simulink model "Full_Model_R1"  (R2013a)
settings: Solver=ode45  StartTime=0.0  StopTime=sim_length  MaxStep=1e-4  RelTol=1e-3
values from neighbouring files (symbols this model uses):
  K = [1 1.29039130411 0.306791381023]    [Yaw_Controller_SS_Data.mat]
  Kp_Height = 3.52780854887    [Height_Controller.mat]
undefined symbols (not defined in the file or in its folder): B, D, F_yIntercept, g, I_Phi, I_Psi, I_Theta, J, Kf, Kw, L, Mass, Motor_TimeConstant, Nbar1, Phi_IC, Pitch_Setpoint, Psi_IC, PWM_LimHigher, PWM_LimLower, Roll_Setpoint, Speed_yIntercept, T_I_Height, Theta_IC, Yaw_Setpoint
libraries: simulink x4
settings Model: Creator=Ross  LastModifiedBy=Ross

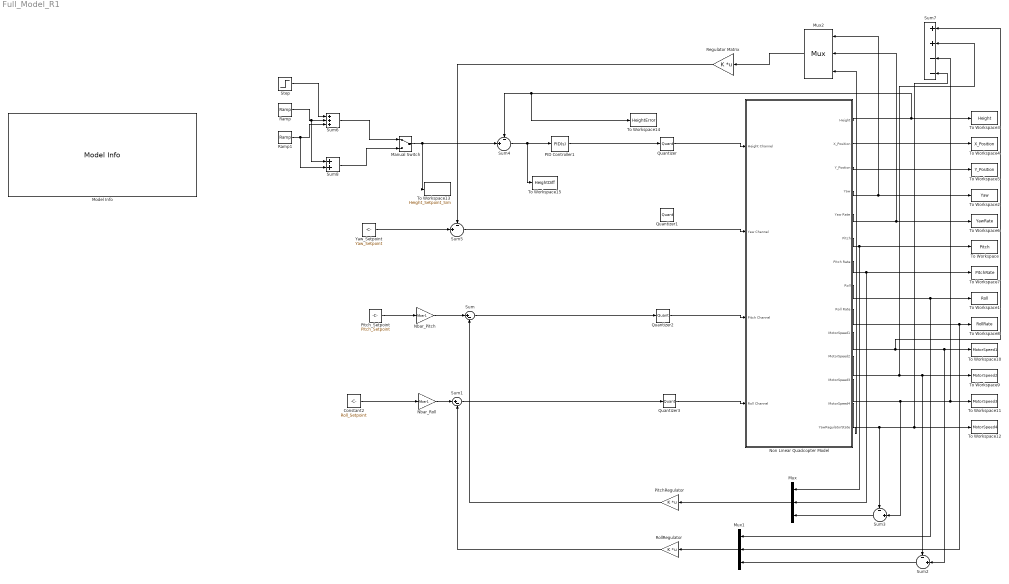
== system Full_Model_R1 ==
  Constant2 : Constant  Value=Roll_Setpoint
  Manual Switch : ManualSwitch
  Model Info : simulink/Model-Wide Utilities/Model Info  InitialBlockCM=None  BlockCM=None  Frame=on  DisplayStringWithTags=|  HorizontalTextAlignment=Center  LeftAlignmentValue=0.5  SourceBlockDiagram=Full_Model_R1  TagMaxNumber=20
      | %<ModelName>
      | Simulink Diagram Used in Testing of Controllers designed for Quadcopters
      | Model version is %<ModelVersion>
      | 
      | %<Created>
      | %<ModifiedBy>
      | %<ModifiedDate>
      | %<ModifiedComment>
      | 
      | 
      | %<LastModifiedBy>
      | %<LastModificationDate>
      | %<Description>
  Mux : Mux  Inputs=3
  Mux1 : Mux  Inputs=3
  Mux2 : Mux  Inputs=3
      settings: DisplayOption=signals
  Nbar_Pitch : Gain  Gain=Nbar1
  Nbar_Roll : Gain  Gain=Nbar1
  Non Linear Quadcopter Model : Subsystem
  PID Controller1 : simulink/Continuous/PID Controller  Controller=PID  TimeDomain=Continuous-time  SampleTime=1  IntegratorMethod=Forward Euler  FilterMethod=Forward Euler  Form=Ideal  P=Kp_Height  I=1/T_I_Height  D=T_I_Height/4  N=100  InitialConditionSource=internal  InitialConditionForIntegrator=0  InitialConditionForFilter=0  ExternalReset=none  LimitOutput=on  UpperSaturationLimit=PWM_LimHigher  LowerSaturationLimit=PWM_LimLower  LinearizeAsGain=on  AntiWindupMode=clamping  Kb=1  TrackingMode=off  Kt=1  PParamMin=[]  PParamMax=[]  IParamMin=[]  IParamMax=[]  DParamMin=[]  DParamMax=[]  NParamMin=[]  NParamMax=[]  KbParamMin=[]  KbParamMax=[]  KtParamMin=[]  KtParamMax=[]  POutMin=[]  POutMax=[]  IOutMin=[]  IOutMax=[]  DOutMin=[]  DOutMax=[]  NOutMin=[]  NOutMax=[]  KbOutMin=[]  KbOutMax=[]  KtOutMin=[]  KtOutMax=[]  IntegratorOutMin=[]  IntegratorOutMax=[]  FilterOutMin=[]  FilterOutMax=[]  SumOutMin=[]  SumOutMax=[]  SumI1OutMin=[]  SumI1OutMax=[]  SumI2OutMin=[]  SumI2OutMax=[]  SumI3OutMin=[]  SumI3OutMax=[]  SumDOutMin=[]  SumDOutMax=[]  SaturationOutMin=[]  SaturationOutMax=[]  IntegratorContinuousStateAttributes=''  IntegratorStateMustResolveToSignalObject=off  IntegratorRTWStateStorageClass=Auto  FilterContinuousStateAttributes=''  FilterStateMustResolveToSignalObject=off  FilterRTWStateStorageClass=Auto
  PitchRegulator : Gain  Gain=K  Multiplication=Matrix(K*u)
  "Pitch_Setpoint " : Constant  Value=Pitch_Setpoint
  Quantizer{,1..3} (4 alike) : Quantizer  QuantizationInterval=8.2e-3  SampleTime=0.02
  Ramp : simulink/Sources/Ramp  slope=1  start=2  X0=0
  Ramp1 : simulink/Sources/Ramp  slope=-1  start=5  X0=0
  Regulator Matrix : Gain  Gain=K  Multiplication=Matrix(K*u)
  RollRegulator : Gain  Gain=K  Multiplication=Matrix(K*u)
  Step : Step  Time=10  SampleTime=0
  Sum : Sum  Inputs=|+-
  Sum1 : Sum  Inputs=|+-
  Sum{2..5} (4 alike) : Sum  Inputs=-|+||
  Sum6 : Sum  Inputs=+++
  Sum7 : Sum  Inputs=++--
  Sum8 : Sum
  To Workspace : ToWorkspace  VariableName=Pitch  SampleTime=-1  SaveFormat=Timeseries
  To Workspace1 : ToWorkspace  VariableName=Roll  SampleTime=-1  SaveFormat=Timeseries
  To Workspace10 : ToWorkspace  VariableName=MotorSpeed1  SampleTime=-1  SaveFormat=Timeseries
  To Workspace11 : ToWorkspace  VariableName=MotorSpeed3  SampleTime=-1  SaveFormat=Timeseries
  To Workspace12 : ToWorkspace  VariableName=MotorSpeed4  SampleTime=-1  SaveFormat=Timeseries
  To Workspace13 : ToWorkspace  VariableName=Height_Setpoint_Sim  SampleTime=-1  SaveFormat=Timeseries
  To Workspace14 : ToWorkspace  VariableName=HeightError  SampleTime=-1  SaveFormat=Timeseries
  To Workspace15 : ToWorkspace  VariableName=HeightDiff  SampleTime=-1  SaveFormat=Timeseries
  To Workspace2 : ToWorkspace  VariableName=Yaw  SampleTime=-1  SaveFormat=Timeseries
  To Workspace3 : ToWorkspace  VariableName=Height  SampleTime=-1  SaveFormat=Timeseries
  To Workspace4 : ToWorkspace  VariableName=X_Position  SampleTime=-1  SaveFormat=Timeseries
  To Workspace5 : ToWorkspace  VariableName=Y_Position  SampleTime=-1  SaveFormat=Timeseries
  To Workspace6 : ToWorkspace  VariableName=YawRate  SampleTime=-1  SaveFormat=Timeseries
  To Workspace7 : ToWorkspace  VariableName=PitchRate  SampleTime=-1  SaveFormat=Timeseries
  To Workspace8 : ToWorkspace  VariableName=RollRate  SampleTime=-1  SaveFormat=Timeseries
  To Workspace9 : ToWorkspace  VariableName=MotorSpeed2  SampleTime=-1  SaveFormat=Timeseries
  Yaw_Setpoint : Constant  Value=Yaw_Setpoint
  wires:
  Sum/1 -> Quantizer2/1
  Sum1/1 -> Quantizer3/1
  Non Linear Quadcopter Model/6(Pitch) -> To Workspace/1, Mux/1
  Non Linear Quadcopter Model/8(Roll) -> Mux1/1, To Workspace1/1
  Non Linear Quadcopter Model/4(Yaw) -> Mux2/1, To Workspace2/1
  Non Linear Quadcopter Model/1(Height) -> To Workspace3/1, To Workspace14/1, Sum4/1
  Non Linear Quadcopter Model/2(X_Position) -> To Workspace4/1
  Non Linear Quadcopter Model/3(Y_Postion) -> To Workspace5/1
  RollRegulator/1 -> Sum1/2
  Nbar_Roll/1 -> Sum1/1
  Nbar_Pitch/1 -> Sum/1
  PitchRegulator/1 -> Sum/2
  "Pitch_Setpoint "/1 -> Nbar_Pitch/1
  Constant2/1 -> Nbar_Roll/1
  Non Linear Quadcopter Model/5(Yaw Rate) -> Mux2/2, To Workspace6/1
  Non Linear Quadcopter Model/7(Pitch Rate) -> To Workspace7/1, Mux/2
  Non Linear Quadcopter Model/9(Roll Rate) -> Mux1/2, To Workspace8/1
  Non Linear Quadcopter Model/10(MotorSpeed1) -> Sum7/1, Sum2/2, To Workspace10/1
  Non Linear Quadcopter Model/11(MotorSpeed2) -> Sum7/2, Sum2/1, To Workspace9/1
  Non Linear Quadcopter Model/12(MotorSpeed3) -> Sum7/3, To Workspace11/1, Sum3/2
  Non Linear Quadcopter Model/13(MotorSpeed4) -> Sum3/1, Sum7/4, To Workspace12/1
  Mux/1 -> PitchRegulator/1
  Sum3/1 -> Mux/3
  Mux1/1 -> RollRegulator/1
  Sum2/1 -> Mux1/3
  Sum4/1 -> To Workspace15/1, PID Controller1/1
  Yaw_Setpoint/1 -> Sum5/2
  PID Controller1/1 -> Quantizer/1
  Ramp/1 -> Sum8/1, Sum6/2
  Ramp1/1 -> Sum8/2, Sum6/3
  Mux2/1 -> Regulator Matrix/1
  Regulator Matrix/1 -> Sum5/1
  Step/1 -> Sum6/1
  Manual Switch/1 -> To Workspace13/1, Sum4/2
  Sum8/1 -> Manual Switch/2
  Sum6/1 -> Manual Switch/1
  Quantizer/1 -> Non Linear Quadcopter Model/1(Height Channel)
  Sum5/1 -> Non Linear Quadcopter Model/2(Yaw Channel)
  Quantizer2/1 -> Non Linear Quadcopter Model/3(Pitch Channel)
  Quantizer3/1 -> Non Linear Quadcopter Model/4(Roll Channel)
  Non Linear Quadcopter Model/14(YawRegulatorState) -> Mux2/3

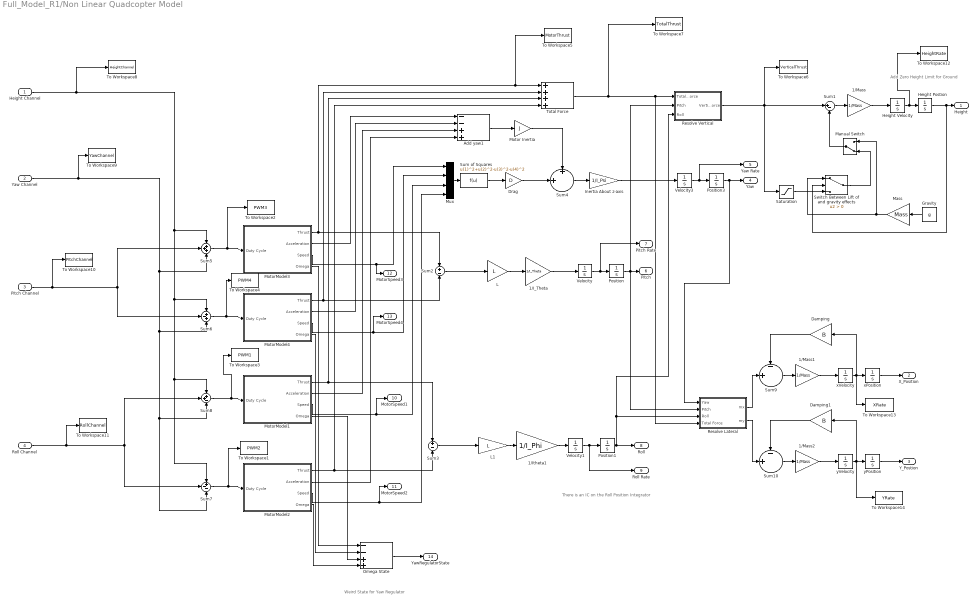
== system Full_Model_R1/Non Linear Quadcopter Model ==
  note: Weird State for Yaw
      | Regulator
  note: There is an IC on the Roll
      | Position Integrator
  note: Add Zero Height Limit
      | for Ground
  Height Channel : Inport
  Yaw Channel : Inport  Port=2
  Pitch Channel : Inport  Port=3
  Roll Channel : Inport  Port=4
  1/I_Theta : Gain  Gain=1/I_Theta
  1/Itheta1 : Gain  Gain=1/I_Phi
  1/Mass : Gain  Gain=1/Mass
  1/Mass1 : Gain  Gain=1/Mass
  1/Mass2 : Gain  Gain=1/Mass
  Add yaw1 : Sum  Inputs=--++
  Damping : Gain  Gain=B
  Damping1 : Gain  Gain=B
  Drag : Gain  Gain=D
  Gravity : Constant  Value=g
  Height Postion : Integrator  LowerSaturationLimit=0
  Height Velocity : Integrator
  Inertia About z-axis : Gain  Gain=1/I_Psi
  L : Gain  Gain=L
  L1 : Gain  Gain=L
  Manual Switch : ManualSwitch  CurrentSetting=0
  Mass : Gain  Gain=Mass
  Motor Inertia : Gain  Gain=J
  MotorModel1 : Subsystem
  MotorModel2 : Subsystem
  MotorModel3 : Subsystem
  MotorModel4 : Subsystem
  Mux : Mux
  Omega State : Sum  Inputs=--++
  Position : Integrator  InitialCondition=Theta_IC
  Position1 : Integrator  InitialCondition=Phi_IC
  Position3 : Integrator  InitialCondition=Psi_IC
  Resolve Lateral : Subsystem
  Resolve Vertical : Subsystem
  Saturation : Saturate  UpperLimit=Mass*g  LowerLimit=-inf
  Sum of Squares : Fcn  Expr=u(1)^2+u(2)^2-u(3)^2-u(4)^2
  Sum1 : Sum  Inputs=|+-
  Sum10 : Sum  Inputs=-|||+||||
  Sum2 : Sum  Inputs=+|-
  Sum3 : Sum  Inputs=+|-
  Sum4 : Sum  Inputs=+|||+||||
  Sum5 : Sum  Inputs=+++
  Sum6 : Sum  Inputs=+-+
  Sum7 : Sum  Inputs=+--
  Sum8 : Sum  Inputs=++-
  Sum9 : Sum  Inputs=-|||+||||
  Switch Between Lift of and gravity effects : Switch  Criteria=u2 > Threshold
  To Workspace1 : ToWorkspace  VariableName=PWM2  SampleTime=-1  SaveFormat=Timeseries
  To Workspace10 : ToWorkspace  VariableName=PitchChannel  SampleTime=-1  SaveFormat=Timeseries
  To Workspace11 : ToWorkspace  VariableName=RollChannel  SampleTime=-1  SaveFormat=Timeseries
  To Workspace12 : ToWorkspace  VariableName=HeightRate  SampleTime=-1  SaveFormat=Timeseries
  To Workspace13 : ToWorkspace  VariableName=XRate  SampleTime=-1  SaveFormat=Timeseries
  To Workspace14 : ToWorkspace  VariableName=YRate  SampleTime=-1  SaveFormat=Timeseries
  To Workspace2 : ToWorkspace  VariableName=PWM3  SampleTime=-1  SaveFormat=Timeseries
  To Workspace3 : ToWorkspace  VariableName=PWM1  SampleTime=-1  SaveFormat=Timeseries
  To Workspace4 : ToWorkspace  VariableName=PWM4  SampleTime=-1  SaveFormat=Timeseries
  To Workspace5 : ToWorkspace  VariableName=MotorThrust  SampleTime=-1  SaveFormat=Timeseries
  To Workspace6 : ToWorkspace  VariableName=VerticalThrust  SampleTime=-1  SaveFormat=Timeseries
  To Workspace7 : ToWorkspace  VariableName=TotalThrust  SampleTime=-1  SaveFormat=Timeseries
  To Workspace8 : ToWorkspace  VariableName=HeightChannel  SampleTime=-1  SaveFormat=Timeseries
  To Workspace9 : ToWorkspace  VariableName=YawChannel  SampleTime=-1  SaveFormat=Timeseries
  Total Force : Sum  Inputs=++++
  Velocity : Integrator
  Velocity1 : Integrator
  Velocity3 : Integrator
  xPosition : Integrator
  xVelocity : Integrator
  yPosition : Integrator
  yVelocity : Integrator
  Height : Outport
  X_Position : Outport  Port=2
  Y_Postion : Outport  Port=3
  Yaw : Outport  Port=4
  Yaw Rate : Outport  Port=5
  Pitch : Outport  Port=6
  Pitch Rate : Outport  Port=7
  Roll : Outport  Port=8
  Roll Rate : Outport  Port=9
  MotorSpeed1 : Outport  Port=10
  MotorSpeed2 : Outport  Port=11
  MotorSpeed3 : Outport  Port=12
  MotorSpeed4 : Outport  Port=13
  YawRegulatorState : Outport  Port=14
  wires:
  Sum1/1 -> 1/Mass/1
  Pitch Channel/1 -> Sum6/2, Sum5/2, To Workspace10/1
  Add yaw1/1 -> Motor Inertia/1
  1/Mass/1 -> Height Velocity/1
  Motor Inertia/1 -> Sum4/1
  1/Mass1/1 -> xVelocity/1
  Sum9/1 -> 1/Mass1/1
  xPosition/1 -> X_Position/1
  Damping/1 -> Sum9/1
  xVelocity/1 -> To Workspace13/1, Damping/1, xPosition/1
  MotorModel3/2(Acceleration) -> Add yaw1/1
  Sum8/1 -> To Workspace3/1, MotorModel1/1(Duty Cycle)
  Height Velocity/1 -> To Workspace12/1, Height Postion/1
  Sum2/1 -> L/1
  1/I_Theta/1 -> Velocity/1
  Velocity/1 -> Pitch Rate/1, Position/1
  Position/1 -> Resolve Vertical/2(Pitch), Pitch/1, Resolve Lateral/2(Pitch)
  Total Force/1 -> To Workspace7/1, Resolve Lateral/4(Total Force), Resolve Vertical/1(Total Force)
  Sum of Squares/1 -> Drag/1
  Drag/1 -> Sum4/2
  Position3/1 -> Yaw/1, Resolve Lateral/1(Yaw)
  Velocity3/1 -> Yaw Rate/1, Position3/1
  Inertia About z-axis/1 -> Velocity3/1
  MotorModel2/1(Thrust) -> Total Force/4, Sum3/2
  L1/1 -> 1/Itheta1/1
  Velocity1/1 -> Roll Rate/1, Position1/1
  Sum3/1 -> L1/1
  Position1/1 -> Roll/1, Resolve Lateral/3(Roll), Resolve Vertical/3(Roll)
  1/Itheta1/1 -> Velocity1/1
  MotorModel3/1(Thrust) -> Sum2/1, To Workspace5/1, Total Force/1
  Sum10/1 -> 1/Mass2/1
  1/Mass2/1 -> yVelocity/1
  yPosition/1 -> Y_Postion/1
  Damping1/1 -> Sum10/1
  yVelocity/1 -> Damping1/1, To Workspace14/1, yPosition/1
  Height Postion/1 -> Switch Between Lift of and gravity effects/2, Height/1
  Sum7/1 -> To Workspace1/1, MotorModel2/1(Duty Cycle)
  MotorModel1/2(Acceleration) -> Add yaw1/3
  MotorModel4/1(Thrust) -> Sum2/2, Total Force/2
  Sum4/1 -> Inertia About z-axis/1
  MotorModel1/1(Thrust) -> Sum3/1, Total Force/3
  Height Channel/1 -> To Workspace8/1, Sum6/1, Sum7/1, Sum8/1, Sum5/1
  Yaw Channel/1 -> To Workspace9/1, Sum7/3, Sum8/3, Sum6/3, Sum5/3
  MotorModel4/2(Acceleration) -> Add yaw1/2
  MotorModel2/2(Acceleration) -> Add yaw1/4
  Sum5/1 -> To Workspace2/1, MotorModel3/1(Duty Cycle)
  Roll Channel/1 -> To Workspace11/1, Sum8/2, Sum7/2
  Gravity/1 -> Mass/1
  Resolve Lateral/1(mx) -> Sum9/2
  Resolve Lateral/2(my) -> Sum10/2
  MotorModel3/3(Speed) -> MotorSpeed3/1, Mux/1
  MotorModel4/3(Speed) -> Mux/2, MotorSpeed4/1
  MotorModel1/3(Speed) -> Mux/3, MotorSpeed1/1
  MotorModel2/3(Speed) -> MotorSpeed2/1, Mux/4
  Mux/1 -> Sum of Squares/1
  L/1 -> 1/I_Theta/1
  Switch Between Lift of and gravity effects/1 -> Manual Switch/2
  Saturation/1 -> Switch Between Lift of and gravity effects/3
  Mass/1 -> Manual Switch/1, Switch Between Lift of and gravity effects/1
  Sum6/1 -> To Workspace4/1, MotorModel4/1(Duty Cycle)
  Manual Switch/1 -> Sum1/2
  Resolve Vertical/1(Vertical Force) -> Sum1/1, Saturation/1, To Workspace6/1
  MotorModel3/4(Omega) -> Omega State/1
  MotorModel4/4(Omega) -> Omega State/2
  MotorModel1/4(Omega) -> Omega State/3
  MotorModel2/4(Omega) -> Omega State/4
  Omega State/1 -> YawRegulatorState/1

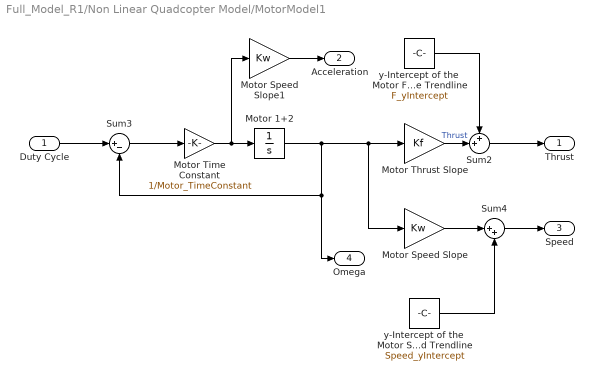
== system Full_Model_R1/Non Linear Quadcopter Model/MotorModel1 ==
  Duty Cycle : Inport
  Motor 1+2 : Integrator
  Motor Speed Slope : Gain  Gain=Kw
  Motor Speed Slope1 : Gain  Gain=Kw
  Motor Thrust Slope : Gain  Gain=Kf
  Motor Time Constant : Gain  Gain=1/Motor_TimeConstant
  Sum2 : Sum  Inputs=++|
  Sum3 : Sum  Inputs=|+-
  Sum4 : Sum  Inputs=|++
  y-Intercept of the  Motor Force Trendline : Constant  Value=F_yIntercept
  y-Intercept of the  Motor Speed Trendline : Constant  Value=Speed_yIntercept
  Thrust : Outport
  Acceleration : Outport  Port=2
  Speed : Outport  Port=3
  Omega : Outport  Port=4
  wires:
  Motor Thrust Slope/1 -> Sum2/2  "Thrust"
  Motor 1+2/1 -> Omega/1, Sum3/2, Motor Speed Slope/1, Motor Thrust Slope/1
  Duty Cycle/1 -> Sum3/1
  Sum3/1 -> Motor Time Constant/1
  Motor Time Constant/1 -> Motor 1+2/1, Motor Speed Slope1/1
  Motor Speed Slope/1 -> Sum4/1
  Motor Speed Slope1/1 -> Acceleration/1
  Sum2/1 -> Thrust/1
  y-Intercept of the  Motor Force Trendline/1 -> Sum2/1
  Sum4/1 -> Speed/1
  y-Intercept of the  Motor Speed Trendline/1 -> Sum4/2

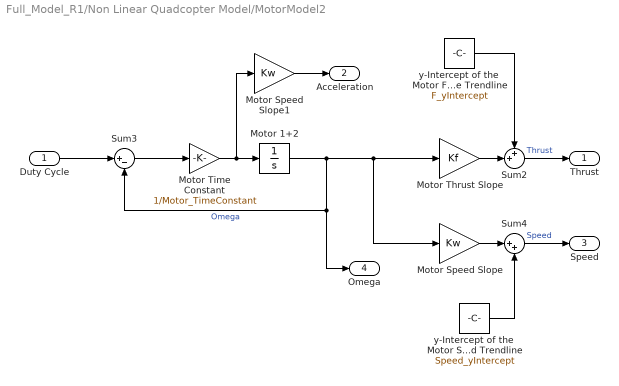
== system Full_Model_R1/Non Linear Quadcopter Model/MotorModel2 ==
  Duty Cycle : Inport
  Motor 1+2 : Integrator
  Motor Speed Slope : Gain  Gain=Kw
  Motor Speed Slope1 : Gain  Gain=Kw
  Motor Thrust Slope : Gain  Gain=Kf
  Motor Time Constant : Gain  Gain=1/Motor_TimeConstant
  Sum2 : Sum  Inputs=++|
  Sum3 : Sum  Inputs=|+-
  Sum4 : Sum  Inputs=|++
  y-Intercept of the  Motor Force Trendline : Constant  Value=F_yIntercept
  y-Intercept of the  Motor Speed Trendline : Constant  Value=Speed_yIntercept
  Thrust : Outport
  Acceleration : Outport  Port=2
  Speed : Outport  Port=3
  Omega : Outport  Port=4
  wires:
  Motor Thrust Slope/1 -> Sum2/2
  Motor 1+2/1 -> Sum3/2, Omega/1, Motor Speed Slope/1, Motor Thrust Slope/1  "Omega"
  Duty Cycle/1 -> Sum3/1
  Sum3/1 -> Motor Time Constant/1
  Motor Time Constant/1 -> Motor 1+2/1, Motor Speed Slope1/1
  Motor Speed Slope/1 -> Sum4/1
  Motor Speed Slope1/1 -> Acceleration/1
  Sum2/1 -> Thrust/1  "Thrust"
  y-Intercept of the  Motor Force Trendline/1 -> Sum2/1
  Sum4/1 -> Speed/1  "Speed"
  y-Intercept of the  Motor Speed Trendline/1 -> Sum4/2

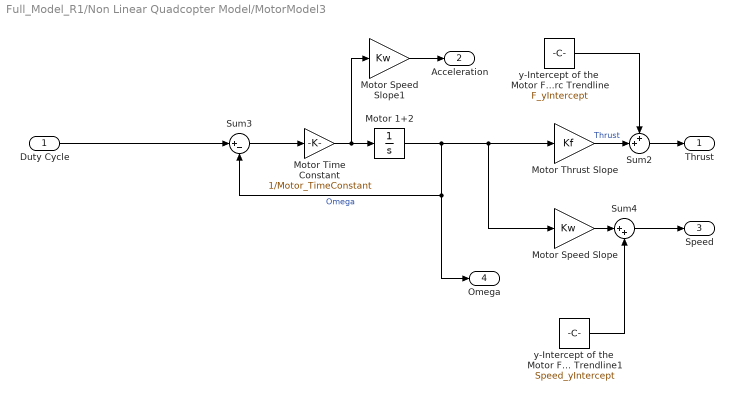
== system Full_Model_R1/Non Linear Quadcopter Model/MotorModel3 ==
  Duty Cycle : Inport
  Motor 1+2 : Integrator
  Motor Speed Slope : Gain  Gain=Kw
  Motor Speed Slope1 : Gain  Gain=Kw
  Motor Thrust Slope : Gain  Gain=Kf
  Motor Time Constant : Gain  Gain=1/Motor_TimeConstant
  Sum2 : Sum  Inputs=++|
  Sum3 : Sum  Inputs=|+-
  Sum4 : Sum  Inputs=|++
  y-Intercept of the  Motor Forc Trendline : Constant  Value=F_yIntercept
  y-Intercept of the  Motor Forc Trendline1 : Constant  Value=Speed_yIntercept
  Thrust : Outport
  Acceleration : Outport  Port=2
  Speed : Outport  Port=3
  Omega : Outport  Port=4
  wires:
  Motor Thrust Slope/1 -> Sum2/2  "Thrust"
  Motor 1+2/1 -> Omega/1, Sum3/2, Motor Speed Slope/1, Motor Thrust Slope/1  "Omega"
  Duty Cycle/1 -> Sum3/1
  Sum3/1 -> Motor Time Constant/1
  Motor Time Constant/1 -> Motor 1+2/1, Motor Speed Slope1/1
  Motor Speed Slope/1 -> Sum4/1
  Motor Speed Slope1/1 -> Acceleration/1
  Sum2/1 -> Thrust/1
  y-Intercept of the  Motor Forc Trendline/1 -> Sum2/1
  Sum4/1 -> Speed/1
  y-Intercept of the  Motor Forc Trendline1/1 -> Sum4/2

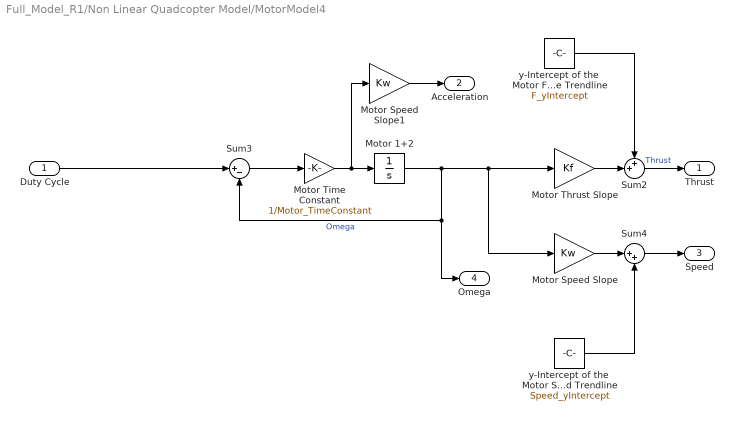
== system Full_Model_R1/Non Linear Quadcopter Model/MotorModel4 ==
  Duty Cycle : Inport
  Motor 1+2 : Integrator
  Motor Speed Slope : Gain  Gain=Kw
  Motor Speed Slope1 : Gain  Gain=Kw
  Motor Thrust Slope : Gain  Gain=Kf
  Motor Time Constant : Gain  Gain=1/Motor_TimeConstant
  Sum2 : Sum  Inputs=++|
  Sum3 : Sum  Inputs=|+-
  Sum4 : Sum  Inputs=|++
  y-Intercept of the  Motor Force Trendline : Constant  Value=F_yIntercept
  y-Intercept of the  Motor Speed Trendline : Constant  Value=Speed_yIntercept
  Thrust : Outport
  Acceleration : Outport  Port=2
  Speed : Outport  Port=3
  Omega : Outport  Port=4
  wires:
  Motor Thrust Slope/1 -> Sum2/2
  Motor 1+2/1 -> Omega/1, Sum3/2, Motor Speed Slope/1, Motor Thrust Slope/1  "Omega"
  Duty Cycle/1 -> Sum3/1
  Sum3/1 -> Motor Time Constant/1
  Motor Time Constant/1 -> Motor 1+2/1, Motor Speed Slope1/1
  Motor Speed Slope/1 -> Sum4/1
  Motor Speed Slope1/1 -> Acceleration/1
  Sum2/1 -> Thrust/1  "Thrust"
  y-Intercept of the  Motor Force Trendline/1 -> Sum2/1
  Sum4/1 -> Speed/1
  y-Intercept of the  Motor Speed Trendline/1 -> Sum4/2

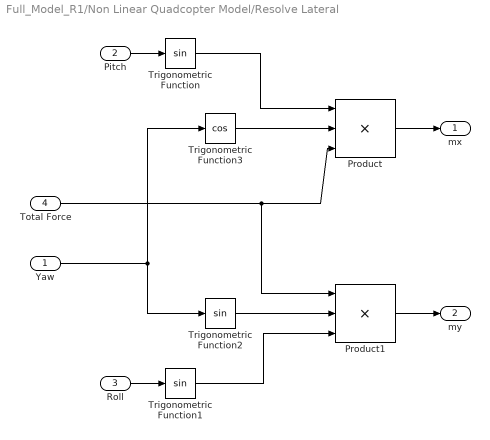
== system Full_Model_R1/Non Linear Quadcopter Model/Resolve Lateral ==
  Yaw : Inport
  Pitch : Inport  Port=2
  Roll : Inport  Port=3
  Total Force : Inport  Port=4
  Product : Product  Inputs=3
  Product1 : Product  Inputs=3
  Trigonometric Function : Trigonometry
  Trigonometric Function1 : Trigonometry
  Trigonometric Function2 : Trigonometry
  Trigonometric Function3 : Trigonometry  Operator=cos
  mx : Outport
  my : Outport  Port=2
  wires:
  Trigonometric Function/1 -> Product/1
  Total Force/1 -> Product1/1, Product/3
  Product/1 -> mx/1
  Roll/1 -> Trigonometric Function1/1
  Trigonometric Function1/1 -> Product1/3
  Product1/1 -> my/1
  Trigonometric Function3/1 -> Product/2
  Trigonometric Function2/1 -> Product1/2
  Yaw/1 -> Trigonometric Function2/1, Trigonometric Function3/1
  Pitch/1 -> Trigonometric Function/1

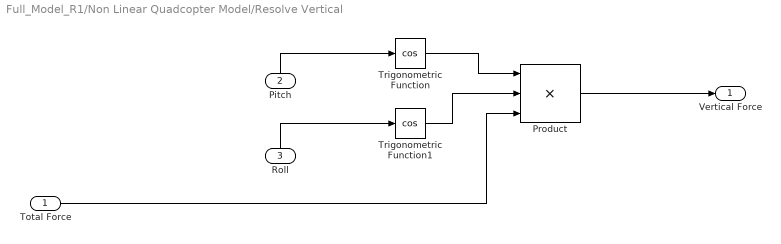
== system Full_Model_R1/Non Linear Quadcopter Model/Resolve Vertical ==
  Total Force : Inport
  Pitch : Inport  Port=2
  Roll : Inport  Port=3
  Product : Product  Inputs=3
  Trigonometric Function : Trigonometry  Operator=cos
  Trigonometric Function1 : Trigonometry  Operator=cos
  Vertical Force : Outport
  wires:
  Trigonometric Function/1 -> Product/1
  Total Force/1 -> Product/3
  Roll/1 -> Trigonometric Function1/1
  Pitch/1 -> Trigonometric Function/1
  Product/1 -> Vertical Force/1
  Trigonometric Function1/1 -> Product/2
